simulink subsystem "PD_controller"  (R2022b)
settings: Solver=VariableStepAuto  StartTime=0.0  StopTime=10.0  RelTol=1e-3
values from neighbouring files (symbols this model uses):
  kd = params.kd    [AME556_HW3_Cornwell.m]    (also in AME_556_Final_Project.m = 4)
  kp = params.kp    [AME556_HW3_Cornwell.m]    (also in AME_556_Final_Project.m = 25)
settings Model: Creator=taracornwell  LastModifiedBy=taracornwell

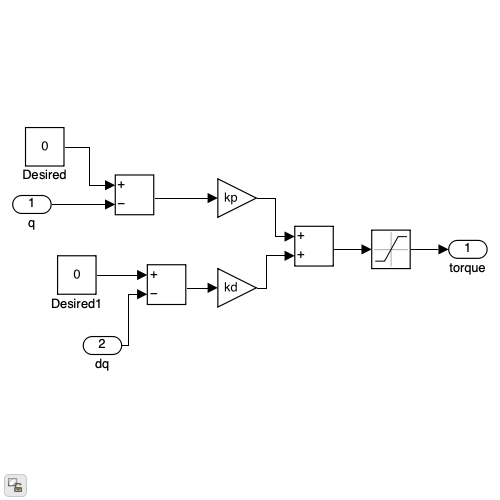
[thumbnail: Simulink's stored preview of the top-level diagram]
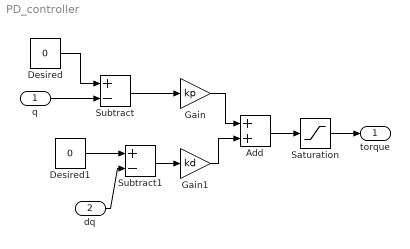
== system PD_controller ==
  q : Inport
  dq : Inport  Port=2
  Add : Sum
  Desired : Constant  Value=0
  Desired1 : Constant  Value=0
  Gain : Gain  Gain=kp
  Gain1 : Gain  Gain=kd
  Saturation : Saturate  UpperLimit=33.5  LowerLimit=-33.5
  Subtract : Sum  Inputs=+-
  Subtract1 : Sum  Inputs=+-
  torque : Outport
  wires:
  Subtract/1 -> Gain/1
  Gain/1 -> Add/1
  Gain1/1 -> Add/2
  Add/1 -> Saturation/1
  Saturation/1 -> torque/1
  q/1 -> Subtract/2
  Desired/1 -> Subtract/1
  Subtract1/1 -> Gain1/1
  Desired1/1 -> Subtract1/1
  dq/1 -> Subtract1/2
